simulink model "MSZSZ_ERR"  (R2025a)
settings: Solver=VariableStepAuto  StartTime=0.0  StopTime=10.0  MaxStep=tau/25  RelTol=1e-3
InitFcn:
  | K = 10;
  | tau = 500e-3;
  | 
  | y_0 = -2;
settings Model: Creator=Szalay  LastModifiedBy=Szalay

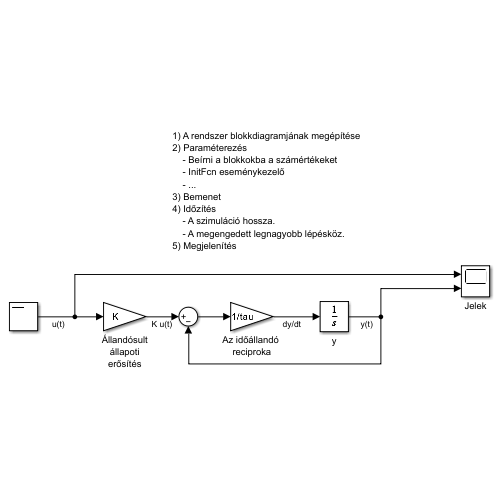
[thumbnail: Simulink's stored preview of the top-level diagram]
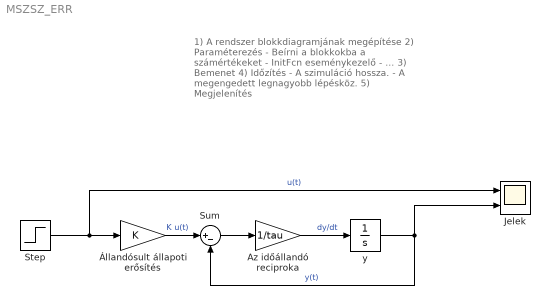
== system MSZSZ_ERR ==
  note: 1) A rendszer blokkdiagramjának megépítése
      | 2) Paraméterezés
      | - Beírni a blokkokba a számértékeket
      | - InitFcn eseménykezelő
      | - ...
      | 3) Bemenet
      | 4) Időzítés
      | - A szimuláció hossza.
      | - A megengedett legnagyobb lépésköz.
      | 5) Megjelenítés
  Az időállandó reciproka : Gain  Gain=1/tau
  Jelek : Scope  NumInputPorts=2
      settings: ActiveDisplayYMinimum=-10.341704146160767  ActiveDisplayYMaximum=1.1490782384623073
  Step : Step  Time=5  After=-1  SampleTime=0
  Sum : Sum  Inputs=|+-
  y : Integrator  InitialCondition=y_0
  Állandósult állapoti erősítés : Gain  Gain=K
  wires:
  y/1 -> Jelek/2, Sum/2  "y(t)"
  Az időállandó reciproka/1 -> y/1  "dy/dt"
  Sum/1 -> Az időállandó reciproka/1
  Állandósult állapoti erősítés/1 -> Sum/1  "K u(t)"
  Step/1 -> Jelek/1, Állandósult állapoti erősítés/1  "u(t)"
